simulink model "HVDC_VSC_1CPUcore_dcpl"  (Simulink 8.4)
settings: Solver=ode3  SolverMode=SingleTasking  StartTime=0.0  StopTime=70.0  FixedStep=Ts_Power  RelTol=1e-3  AbsTol=1e-2
PreLoadFcn:
  | Ts_Power=50e-6; Ts_Control=1*Ts_Power; init_cosim_IA; startup_transients_hvdc_vsc;
PostLoadFcn:
  | Ts_Power=50e-6; Ts_Control=1*Ts_Power; init_cosim_IA; startup_transients_hvdc_vsc;
InitFcn:
  | Ts_Power=50e-6; Ts_Control=1*Ts_Power; init_cosim_IA; startup_transients_hvdc_vsc;
values from neighbouring files (symbols this model uses):
  h = 5    [init_cosim_IA.m]
  intfDelay = 400.0    (= 400)    [init_cosim_IA.m]
  Ts_intf = 2*Ts_Power    [init_cosim_IA.m]
undefined symbols (not defined in the file or in its folder): CLARK, D1, Delta, dPref1_2, dPref1_2_rlimit, gcbh, level, lib_mesures, magnitude, ResistanceM, rte_drive_private_lib, rte_tsb3level_hiz_rect_cb, sps_rtmsupport, t_deblock_Pref1, t_deblock_Udref2, t_dPref1_2, t_init_AC, t_SwitchITMIdc, t_SwitchITMVdc, t_vsag_end, t_vsag_start, TSB3_hiZR
libraries: powerlib x162, powerlib_extras x71, spsVIMeasurementModel x63, rteventslib x26, op_dpl_lib x14, powerlib_meascontrol x14, rtlab x6, sps_avr x3, artemis x1
(part 7 of 11)

== system HVDC_VSC_1CPUcore_dcpl/SM_HVDC_VSC/VSC Controller (Station 2)/Discrete VSC Controller (Station 2)/Outer Active-Reactive Power and Voltage Loop ==
  note: Outer Active-Reactive Power and Voltage Loop
  Udc_meas : Inport
  Uf_meas : Inport  Port=2
  P_meas : Inport  Port=3
  Q_meas : Inport  Port=4
  U_meas : Inport  Port=5
  Pref : Inport  Port=6
  dPref : Inport  Port=7
  Qref : Inport  Port=8
  Udref : Inport  Port=9
  block_status : Inport  Port=10
  Active_Power_Control : Subsystem
  Constant19 : Constant  Value=Ki_dcvc
  Constant20 : Constant  Value=Kp_dcvc
  Constant9 : Constant  Value=P_control
  Current_Reference_Calculation : Subsystem
  Current_Reference_Limitation : Subsystem
  DC_Voltage_Control : Subsystem  TreatAsAtomicUnit=on
  Logical Operator1 : Logic  AllPortsSameDT=off
  Logical Operator4 : Logic  Operator=NOT  AllPortsSameDT=off
  Logical Operator6 : Logic  AllPortsSameDT=off
  Logical Operator7 : Logic  Operator=NOT  AllPortsSameDT=off
  Reactive_Power_Control : Subsystem
  Switch2 : Switch  Threshold=0.5  SaturateOnIntegerOverflow=on
  Iref_dq : Outport
  Pref_ramped : Outport  Port=2
  wires:
  Current_Reference_Limitation/1(Iref_dq) -> Iref_dq/1
  Switch2/1 -> Current_Reference_Limitation/1(Iref_d_tmp)
  Logical Operator4/1 -> Logical Operator1/1, Logical Operator6/2, Active_Power_Control/2(enable_ramp), Reactive_Power_Control/1(enable_control)
  Current_Reference_Calculation/1(Iref_d_crc) -> Switch2/1
  Constant20/1 -> DC_Voltage_Control/4(Kp_dcvc)
  Constant19/1 -> DC_Voltage_Control/3(Ki_dcvc)
  Q_meas/1 -> Reactive_Power_Control/3(Q_meas)
  P_meas/1 -> Active_Power_Control/5(P_meas)
  DC_Voltage_Control/1(Iref_d_dcvc) -> Switch2/3
  Udc_meas/1 -> Active_Power_Control/7(Udc_meas), DC_Voltage_Control/2(Udc_meas)
  block_status/1 -> Logical Operator4/1
  Constant9/1 -> Logical Operator6/1, Current_Reference_Limitation/3(P_control), Logical Operator7/1
  Logical Operator6/1 -> Switch2/2, Active_Power_Control/1(enable_control)
  U_meas/1 -> Reactive_Power_Control/4(U_meas), Active_Power_Control/6(U_meas)
  Current_Reference_Calculation/2(Iref_q_crc) -> Current_Reference_Limitation/2(Iref_q_tmp)
  dPref/1 -> Active_Power_Control/4(dPref)
  Active_Power_Control/1(Pref_apc) -> Current_Reference_Calculation/1(Pref_apc)
  Reactive_Power_Control/1(Qref_rpc) -> Current_Reference_Calculation/2(Qref_rpc)
  Pref/1 -> Active_Power_Control/3(Pref)
  Uf_meas/1 -> Current_Reference_Calculation/3(Uf_meas)
  Qref/1 -> Reactive_Power_Control/2(Qref)
  Logical Operator7/1 -> Logical Operator1/2
  Logical Operator1/1 -> DC_Voltage_Control/Enable
  Udref/1 -> DC_Voltage_Control/1(Udref)
  Active_Power_Control/2(Pref_ramped) -> Pref_ramped/1

== system HVDC_VSC_1CPUcore_dcpl/SM_HVDC_VSC/VSC Controller (Station 2)/Discrete VSC Controller (Station 2)/PLL ==
  note: Discrete 3-phase PLL
  note: Pierre Giroux, Gilbert Sybille
      | Power System Laboratory, IREQ
      | Hydro-Quebec
  U_AB : Inport
  Constant1 : Constant  Value=0
  Constant4 : Constant  Value=2*pi
  Discrete PI Controller : powerlib_extras/Discrete  Control Blocks/Discrete PI Controller  Kp=Kp  Ki=Ki  Par_Limits=2*pi*Finit*[1.25 0.75]  Init=2*pi*Finit  Ts=Ts
  Discrete Rate Limiter : powerlib_extras/Discrete  Control Blocks/Discrete Rate Limiter  R=12  F=-12  Vinit=Finit  Ts=Ts
  Discrete Variable Frequency Mean value : powerlib_extras/Discrete Measurements/Discrete Variable Frequency Mean value  Finit=Finit  Fmin=Fmin  Vinit=0  Ts=Ts
  Discrete  2nd-Order Filter : powerlib_extras/Discrete  Control Blocks/Discrete  2nd-Order Filter  FilterType=Lowpass  Fo=25  Zeta=0.707  Ts=Ts  Initialize=on  Vac_Init=[0 0 Finit]  Vdc_Init=Finit  PlotResponse=off  param1=[1 500 0.1]
  Discrete-Time Integrator : DiscreteIntegrator  InitialCondition=Phase_Init*pi/180  SampleTime=Ts
  Gain10 : Gain  Gain=1/2/pi  SaturateOnIntegerOverflow=on  OutDataTypeStr=Inherit: Same as input  ParamDataTypeStr=Inherit: Same as input
  Math Function : Math  Operator=mod  SaturateOnIntegerOverflow=on
  Mux1 : Mux  Inputs=[2 1]
  Mux2 : Mux  Inputs=2
  Selector : Selector  InputPortWidth=3  Indices=2
  Trigonometric Function : Trigonometry
  Trigonometric Function2 : Trigonometry  Operator=cos
  Unit Delay : UnitDelay  InitialCondition=Finit  SampleTime=Ts
  "ab0->dq0 " : Subsystem  AncestorBlock=lib_mesures/CLARK
  Freq : Outport
  theta : Outport  Port=2
  Sin_Cos : Outport  Port=3
  wires:
  Constant1/1 -> Mux1/2
  Mux1/1 -> "ab0->dq0 "/1(ab0)
  U_AB/1 -> Mux1/1
  Discrete Variable Frequency Mean value/1 -> Discrete PI Controller/1
  "ab0->dq0 "/1(dq0) -> Selector/1
  Constant4/1 -> Math Function/2
  Discrete-Time Integrator/1 -> Math Function/1
  Math Function/1 -> Trigonometric Function/1, Trigonometric Function2/1, theta/1
  Trigonometric Function/1 -> Mux2/1
  Trigonometric Function2/1 -> Mux2/2
  Mux2/1 -> "ab0->dq0 "/2(sin_cos), Sin_Cos/1
  Discrete PI Controller/1 -> Discrete-Time Integrator/1, Gain10/1  "W"
  Gain10/1 -> Discrete Rate Limiter/1
  Discrete Rate Limiter/1 -> Discrete  2nd-Order Filter/1
  Unit Delay/1 -> Freq/1, Discrete Variable Frequency Mean value/1
  Discrete  2nd-Order Filter/1 -> Unit Delay/1
  Selector/1 -> Discrete Variable Frequency Mean value/2  "Vq"

== system HVDC_VSC_1CPUcore_dcpl/SM_HVDC_VSC/VSC Controller (Station 2)/Discrete VSC Controller (Station 2)/Signal Calculations ==
  U_AB : Inport
  I_AB : Inport  Port=2
  Uf_AB : Inport  Port=3
  Vref_lim_AB : Inport  Port=4
  Udc_pn : Inport  Port=5
  Idc_pn : Inport  Port=6
  Freq : Inport  Port=7
  2nd-Order Filter : powerlib_extras/Discrete  Control Blocks/Discrete  2nd-Order Filter  FilterType=Lowpass  Fo=f0_sc  Zeta=zeta_sc  Ts=Ts_Control  Initialize=off  Vac_Init=[0.8 -25 60]  Vdc_Init=-0.4  PlotResponse=off  param1=[1 500 1]
  2nd-Order Filter2 : powerlib_extras/Discrete  Control Blocks/Discrete  2nd-Order Filter  FilterType=Lowpass  Fo=f0_sc  Zeta=zeta_sc  Ts=Ts_Control  Initialize=off  Vac_Init=[0.8 -25 60]  Vdc_Init=-0.4  PlotResponse=off  param1=[1 500 1]
  "2nd-Order Filter " : powerlib_extras/Discrete  Control Blocks/Discrete  2nd-Order Filter  FilterType=Lowpass  Fo=f0_sc  Zeta=zeta_sc  Ts=Ts_Control  Initialize=off  Vac_Init=[0.8 -25 60]  Vdc_Init=-0.4  PlotResponse=off  param1=[1 500 1]
  "2nd-Order Filter  " : powerlib_extras/Discrete  Control Blocks/Discrete  2nd-Order Filter  FilterType=Lowpass  Fo=f0_sc  Zeta=zeta_sc  Ts=Ts_Control  Initialize=off  Vac_Init=[0.8 -25 60]  Vdc_Init=-0.4  PlotResponse=off  param1=[1 500 1]
  2nd-Order Filter 1\ : powerlib_extras/Discrete  Control Blocks/Discrete  2nd-Order Filter  FilterType=Lowpass  Fo=f0_sc  Zeta=zeta_sc  Ts=Ts_Control  Initialize=off  Vac_Init=[0.8 -25 60]  Vdc_Init=-0.4  PlotResponse=off  param1=[1 500 1]
  Active_Power : Subsystem
  DC_Current : Subsystem
  DC_Voltage : Subsystem
  Demux : Demux  Outputs=2
  Demux1 : Demux  Outputs=2
  Filter_Bus_Voltage : Subsystem
  Gain1 : Gain  Gain=k_pu2nom_Vdc*k_pu2nom_Idc  SaturateOnIntegerOverflow=on  OutDataTypeStr=Inherit: Same as input  ParamDataTypeStr=Inherit: Same as input
  Modulation_Index : Subsystem
  PCC_Voltage : Subsystem
  Product5 : Product  SaturateOnIntegerOverflow=on  OutDataTypeStr=Inherit: Same as first input
  Reactive_Power : Subsystem
  Variable Frequency Mean value IC: 0 : powerlib_extras/Discrete Measurements/Discrete Variable Frequency Mean value  Finit=50  Fmin=f_min_pll  Vinit=0  Ts=Ts_Control
  Pdc_meas : Outport
  Mod_index : Outport  Port=2
  Udc_meas : Outport  Port=3
  Uf_meas : Outport  Port=4
  P_meas : Outport  Port=5
  Q_meas : Outport  Port=6
  U_meas : Outport  Port=7
  wires:
  Gain1/1 -> Pdc_meas/1
  Freq/1 -> Variable Frequency Mean value IC: 0/1
  Product5/1 -> Gain1/1
  Variable Frequency Mean value IC: 0/1 -> Product5/2
  2nd-Order Filter 1\/1 -> Uf_meas/1
  "2nd-Order Filter "/1 -> Mod_index/1
  Filter_Bus_Voltage/1(Uf_meas) -> 2nd-Order Filter 1\/1
  PCC_Voltage/1(Upcc) -> "2nd-Order Filter  "/1
  "2nd-Order Filter  "/1 -> U_meas/1
  Active_Power/1(Ppcc) -> 2nd-Order Filter/1
  2nd-Order Filter/1 -> P_meas/1
  Reactive_Power/1(Qpcc) -> 2nd-Order Filter2/1
  2nd-Order Filter2/1 -> Q_meas/1
  Modulation_Index/1(Mod_index) -> "2nd-Order Filter "/1
  Demux/2 -> DC_Voltage/2(Udc_n)
  Uf_AB/1 -> Filter_Bus_Voltage/1(Uf_AB)
  U_AB/1 -> PCC_Voltage/1(U_AB), Active_Power/1(U_AB), Reactive_Power/1(U_AB)
  I_AB/1 -> Active_Power/2(I_AB), Reactive_Power/2(I_AB)
  DC_Voltage/1(Udc_meas) -> Product5/1, Udc_meas/1, Modulation_Index/2(Udc_meas)
  DC_Current/1(Idc_meas) -> Variable Frequency Mean value IC: 0/2
  Udc_pn/1 -> Demux/1
  Demux/1 -> DC_Voltage/1(Udc_p)
  Demux1/1 -> DC_Current/1(Idc_p)
  Demux1/2 -> DC_Current/2(Idc_n)
  Idc_pn/1 -> Demux1/1
  Vref_lim_AB/1 -> Modulation_Index/1(Vref_lim_AB)

== system HVDC_VSC_1CPUcore_dcpl/SM_HVDC_VSC/VSC Controller (Station 2)/Discrete VSC Controller (Station 2)/dq  Transformations ==
  note: dq Transformations
  U_AB : Inport
  Iv_AB : Inport  Port=2
  sin_cos : Inport  Port=3
  Constant1 : Constant  Value=0
  Mux1 : Mux  Inputs=[2 1]
  Mux4 : Mux  Inputs=[2 1]
  Selector : Selector  InputPortWidth=3  Indices=[1 2]
  Selector3 : Selector  InputPortWidth=3  Indices=[1 2]
  ab0_to_dq0 : Subsystem  AncestorBlock=lib_mesures/CLARK
  "ab0_to_dq0   " : Subsystem  AncestorBlock=lib_mesures/CLARK
  U_dq : Outport
  Iv_dq : Outport  Port=2
  wires:
  Constant1/1 -> Mux4/2, Mux1/2
  Mux4/1 -> "ab0_to_dq0   "/1(ab0)
  Iv_AB/1 -> Mux4/1
  Mux1/1 -> ab0_to_dq0/1(ab0)
  U_AB/1 -> Mux1/1
  "ab0_to_dq0   "/1(dq0) -> Selector3/1
  ab0_to_dq0/1(dq0) -> Selector/1
  sin_cos/1 -> "ab0_to_dq0   "/2(sin_cos), ab0_to_dq0/2(sin_cos)
  Selector/1 -> U_dq/1
  Selector3/1 -> Iv_dq/1

== system HVDC_VSC_1CPUcore_dcpl/SM_HVDC_VSC/VSC Controller (Station 1)/Discrete VSC Controller (Station 1)/Clark Transformations/CLARK  ==
  note: CLARK transformation
  abc : Inport
  Fcn1 : Fcn  Expr=1/sqrt(3)*(u[2] - u[3])
  Fcn2 : Fcn  Expr=1/3*(2*u[1] - u[2] - u[3])
  Fcn3 : Fcn  Expr=1/3*(u[1] + u[2] + u[3])
  Mux : Mux  Inputs=3
  AB0 : Outport
  wires:
  Fcn2/1 -> Mux/1
  abc/1 -> Fcn1/1, Fcn3/1, Fcn2/1
  Fcn1/1 -> Mux/2
  Fcn3/1 -> Mux/3
  Mux/1 -> AB0/1

== system HVDC_VSC_1CPUcore_dcpl/SM_HVDC_VSC/VSC Controller (Station 1)/Discrete VSC Controller (Station 1)/Clark Transformations/CLARK   ==
  note: CLARK transformation
  abc : Inport
  Fcn1 : Fcn  Expr=1/sqrt(3)*(u[2] - u[3])
  Fcn2 : Fcn  Expr=1/3*(2*u[1] - u[2] - u[3])
  Fcn3 : Fcn  Expr=1/3*(u[1] + u[2] + u[3])
  Mux : Mux  Inputs=3
  AB0 : Outport
  wires:
  Mux/1 -> AB0/1
  Fcn3/1 -> Mux/3
  Fcn1/1 -> Mux/2
  abc/1 -> Fcn2/1, Fcn3/1, Fcn1/1
  Fcn2/1 -> Mux/1

== system HVDC_VSC_1CPUcore_dcpl/SM_HVDC_VSC/VSC Controller (Station 1)/Discrete VSC Controller (Station 1)/Clark Transformations/CLARK_YD ==
  note: Rotation of pi/6
  note: Rotation of - pi/6
  note: Transformer Connexion:
      | YY = 0
      | YD1 (laging) = 1
      | YD11 (leading)= 2
  note: CLARK transformation
  abc : Inport
  Tr_conx : Inport  Port=2
  CLARK : Subsystem  AncestorBlock=lib_mesures/CLARK  TreatAsAtomicUnit=on
  CLARK_YD1 : Subsystem  AncestorBlock=lib_mesures/CLARK  TreatAsAtomicUnit=on
  CLARK_YD11 : Subsystem  AncestorBlock=lib_mesures/CLARK  TreatAsAtomicUnit=on
  Constant : Constant  Value=2
  Constant1 : Constant  Value=0
  Constant2 : Constant
  Relational Operator1 : RelationalOperator  Operator===  InputSameDT=on
  Relational Operator2 : RelationalOperator  Operator===  InputSameDT=on
  Relational Operator3 : RelationalOperator  Operator===  InputSameDT=on
  Sum : Sum  Inputs=+++  SaturateOnIntegerOverflow=on
  AB0 : Outport
  wires:
  Constant2/1 -> Relational Operator3/2
  Relational Operator2/1 -> CLARK/Enable
  Constant1/1 -> Relational Operator2/2
  CLARK/1(AB0) -> Sum/3
  Sum/1 -> AB0/1
  CLARK_YD1/1(AB0) -> Sum/2
  CLARK_YD11/1(AB0) -> Sum/1
  abc/1 -> CLARK/1(abc), CLARK_YD1/1(abc), CLARK_YD11/1(abc)
  Relational Operator1/1 -> CLARK_YD11/Enable
  Relational Operator3/1 -> CLARK_YD1/Enable
  Tr_conx/1 -> Relational Operator3/1, Relational Operator2/1, Relational Operator1/1
  Constant/1 -> Relational Operator1/2

== system HVDC_VSC_1CPUcore_dcpl/SM_HVDC_VSC/VSC Controller (Station 1)/Discrete VSC Controller (Station 1)/Clark Transformations/CLARK_YD  ==
  note: CLARK transformation
  note: Transformer Connexion:
      | YY = 0
      | YD1 (laging) = 1
      | YD11 (leading)= 2
  note: Rotation of - pi/6
  note: Rotation of pi/6
  abc : Inport
  Tr_conx : Inport  Port=2
  CLARK : Subsystem  AncestorBlock=lib_mesures/CLARK  TreatAsAtomicUnit=on
  CLARK_YD1 : Subsystem  AncestorBlock=lib_mesures/CLARK  TreatAsAtomicUnit=on
  CLARK_YD11 : Subsystem  AncestorBlock=lib_mesures/CLARK  TreatAsAtomicUnit=on
  Constant : Constant  Value=2
  Constant1 : Constant  Value=0
  Constant2 : Constant
  Relational Operator1 : RelationalOperator  Operator===  InputSameDT=on
  Relational Operator2 : RelationalOperator  Operator===  InputSameDT=on
  Relational Operator3 : RelationalOperator  Operator===  InputSameDT=on
  Sum : Sum  Inputs=+++  SaturateOnIntegerOverflow=on
  AB0 : Outport
  wires:
  Constant/1 -> Relational Operator1/2
  Tr_conx/1 -> Relational Operator1/1, Relational Operator2/1, Relational Operator3/1
  Relational Operator3/1 -> CLARK_YD1/Enable
  Relational Operator1/1 -> CLARK_YD11/Enable
  abc/1 -> CLARK_YD11/1(abc), CLARK_YD1/1(abc), CLARK/1(abc)
  CLARK_YD11/1(AB0) -> Sum/1
  CLARK_YD1/1(AB0) -> Sum/2
  Sum/1 -> AB0/1
  CLARK/1(AB0) -> Sum/3
  Constant1/1 -> Relational Operator2/2
  Relational Operator2/1 -> CLARK/Enable
  Constant2/1 -> Relational Operator3/2

== system HVDC_VSC_1CPUcore_dcpl/SM_HVDC_VSC/VSC Controller (Station 1)/Discrete VSC Controller (Station 1)/DC Voltage Balance Control/Regulator ==
  note: Reset states when enabling
  note: Voltage Sign
  note: Reversed Current Sign
  V_ref_lim_abc : Inport
  Iv_abc : Inport  Port=2
  Udc_0_mean : Inport  Port=3
  Enable : EnablePort  StatesWhenEnabling=reset
  Constant1 : Constant  Value=0
  Constant13 : Constant  Value=Ki_dcvbc
  Constant2 : Constant  Value=0
  Constant3 : Constant  Value=-1
  Constant4 : Constant
  Constant5 : Constant
  Constant6 : Constant  Value=-1
  Constant7 : Constant  Value=0
  Constant8 : Constant  Value=Kp_dcvbc
  "PI_regulator " : Subsystem  mask(PI regulator - type 2){max_i=max_out_dcvbc, min_i=min_out_dcvbc, i_ic=0, max_out=max_out_dcvbc, min_out=min_out_dcvbc, Ts=Ts_Control}
      mask prompts: max_i "Integrator maximum  limit:"; min_i "Integrator minimum  limit:"; i_ic "Integrator initial condition:"; max_out "Output maximum limit:"; min_out "Output minimum limit:"; Ts "Sample time: (s)"
  Product : Product  Inputs=3  SaturateOnIntegerOverflow=on  OutDataTypeStr=Inherit: Same as first input
  Relational Operator : RelationalOperator  Operator=<
  Relational Operator1 : RelationalOperator  Operator=<
  Switch : Switch  Threshold=0.5  SaturateOnIntegerOverflow=on
  Switch1 : Switch  Threshold=0.5  SaturateOnIntegerOverflow=on
  dV_ref_abc_dcvbc : Outport
  wires:
  Switch1/1 -> Product/2
  Constant1/1 -> "PI_regulator "/5(Kf), "PI_regulator "/2(Meas)
  Constant13/1 -> "PI_regulator "/3(Ki)
  Constant8/1 -> "PI_regulator "/4(Kp)
  "PI_regulator "/1(Out) -> Product/3
  Constant2/1 -> Relational Operator/2
  Constant3/1 -> Switch/1
  Constant4/1 -> Switch/3
  Relational Operator/1 -> Switch/2
  Constant5/1 -> Switch1/1
  Constant6/1 -> Switch1/3
  Relational Operator1/1 -> Switch1/2
  Switch/1 -> Product/1
  V_ref_lim_abc/1 -> Relational Operator/1
  Product/1 -> dV_ref_abc_dcvbc/1
  Iv_abc/1 -> Relational Operator1/1
  Udc_0_mean/1 -> "PI_regulator "/1(Ord)
  Constant7/1 -> Relational Operator1/2

== system HVDC_VSC_1CPUcore_dcpl/SM_HVDC_VSC/VSC Controller (Station 1)/Discrete VSC Controller (Station 1)/Inner Current Loop/AC_Current_Control ==
  note: Uq
  note: Ud
  note: AC Current Control
  note: d axis
  note: q axis
  Iv_dq : Inport
  Iref_dq : Inport  Port=2
  U_dq : Inport  Port=3
  Freq : Inport  Port=4
  Constant1 : Constant  Value=Kp_accc
  Constant13 : Constant  Value=Ki_accc
  Constant2 : Constant  Value=1.0
  Constant3 : Constant  Value=Kf_accc
  Demux : Demux  Outputs=2
  Demux1 : Demux  Outputs=2
  Demux2 : Demux  Outputs=2
  IC: 1.0 : powerlib_extras/Discrete Measurements/Discrete Variable Frequency Mean value  Finit=60  Fmin=f_min_pll  Vinit=1.0  Ts=Ts_Control
  Mux : Mux  Inputs=2
  "PI_regulator " : Subsystem  mask(PI regulator - type 2){max_i=max_out_accc, min_i=min_out_accc, i_ic=0, max_out=max_out_accc, min_out=min_out_accc, Ts=Ts_Control}
      mask prompts: max_i "Integrator maximum  limit:"; min_i "Integrator minimum  limit:"; i_ic "Integrator initial condition:"; max_out "Output maximum limit:"; min_out "Output minimum limit:"; Ts "Sample time: (s)"
  PI_regulator_2 : Subsystem  mask(PI regulator - type 2){max_i=max_out_accc, min_i=min_out_accc, i_ic=0, max_out=max_out_accc, min_out=min_out_accc, Ts=Ts_Control}
      mask prompts: max_i "Integrator maximum  limit:"; min_i "Integrator minimum  limit:"; i_ic "Integrator initial condition:"; max_out "Output maximum limit:"; min_out "Output minimum limit:"; Ts "Sample time: (s)"
  Product : Product  SaturateOnIntegerOverflow=on  OutDataTypeStr=Inherit: Same as first input
  Product1 : Product  SaturateOnIntegerOverflow=on  OutDataTypeStr=Inherit: Same as first input
  Sum2 : Sum  Inputs=+|-|+  SaturateOnIntegerOverflow=on  InputSameDT=on  OutDataTypeStr=Inherit: Same as first input
  Sum3 : Sum  Inputs=--+  SaturateOnIntegerOverflow=on  InputSameDT=on  OutDataTypeStr=Inherit: Same as first input
  "Variable Frequency Mean value IC:1.0 " : powerlib_extras/Discrete Measurements/Discrete Variable Frequency Mean value  Finit=60  Fmin=f_min_pll  Vinit=1.0  Ts=Ts_Control
  Vref_dq_tmp : Outport
  wires:
  Constant3/1 -> Product1/1, Product/2
  Sum3/1 -> Mux/2
  IC: 1.0/1 -> Sum3/3
  Demux2/2 -> IC: 1.0/2
  Product1/1 -> Sum3/2
  Sum2/1 -> Mux/1
  "Variable Frequency Mean value IC:1.0 "/1 -> Sum2/1
  Freq/1 -> IC: 1.0/1, "Variable Frequency Mean value IC:1.0 "/1
  Demux2/1 -> "Variable Frequency Mean value IC:1.0 "/2
  Product/1 -> Sum2/3
  PI_regulator_2/1(Out) -> Sum3/1
  "PI_regulator "/1(Out) -> Sum2/2
  Iref_dq/1 -> Demux1/1
  Iv_dq/1 -> Demux/1
  Demux1/1 -> "PI_regulator "/1(Ord)  "I_ref_d"
  Demux/1 -> Product1/2, "PI_regulator "/2(Meas)  "Iv_d"
  Constant2/1 -> "PI_regulator "/5(Kf), PI_regulator_2/5(Kf)
  Demux/2 -> Product/1, PI_regulator_2/2(Meas)  "Iv_q"
  Constant13/1 -> "PI_regulator "/3(Ki), PI_regulator_2/3(Ki)
  Mux/1 -> Vref_dq_tmp/1
  Constant1/1 -> "PI_regulator "/4(Kp), PI_regulator_2/4(Kp)
  Demux1/2 -> PI_regulator_2/1(Ord)  "I_ref_q"
  U_dq/1 -> Demux2/1

== system HVDC_VSC_1CPUcore_dcpl/SM_HVDC_VSC/VSC Controller (Station 1)/Discrete VSC Controller (Station 1)/Inner Current Loop/Inverse_Clark ==
  note: Inverse CLARK transformation
  AB0 : Inport
  Fcn1 : Fcn  Expr="1/2*(-u[1]  + sqrt(3)*u[2] + 2*u[3])"
  Fcn2 : Fcn  Expr=(u[1] - u[3])
  Fcn3 : Fcn  Expr=1/2*(-u[1] - sqrt(3)*u[2] + 2*u[3])
  Mux : Mux  Inputs=3
  abc : Outport
  wires:
  Fcn2/1 -> Mux/1
  AB0/1 -> Fcn1/1, Fcn3/1, Fcn2/1
  Fcn1/1 -> Mux/2
  Fcn3/1 -> Mux/3
  Mux/1 -> abc/1

== system HVDC_VSC_1CPUcore_dcpl/SM_HVDC_VSC/VSC Controller (Station 1)/Discrete VSC Controller (Station 1)/Inner Current Loop/Reference_Voltage_Conditioning ==
  note: Maximum AC Voltage / DC Voltage (pole-neutral)
  note: Voltage Reference Conditioning
  Vref_dq_tmp : Inport
  Udc_meas_mean : Inport  Port=2
  Constant2 : Constant  Value=K_pwm
  Gain1 : Gain  Gain=k_pu2nom_Vdc  SaturateOnIntegerOverflow=on  OutDataTypeStr=Inherit: Same as input  ParamDataTypeStr=Inherit: Same as input
  Product1 : Product  Inputs=**/  SaturateOnIntegerOverflow=on  OutDataTypeStr=Inherit: Same as first input
  Vref_dq : Outport
  wires:
  Gain1/1 -> Product1/2
  Udc_meas_mean/1 -> Gain1/1
  Product1/1 -> Vref_dq/1
  Vref_dq_tmp/1 -> Product1/1
  Constant2/1 -> Product1/3

== system HVDC_VSC_1CPUcore_dcpl/SM_HVDC_VSC/VSC Controller (Station 1)/Discrete VSC Controller (Station 1)/Inner Current Loop/Reference_Voltage_Limitation ==
  note: Limitation on a circle of 1 p.u. radius
  note: Reference Voltage Limitation
  note: Not Limited
  note: Limited
  Vref_dq : Inport
  Constant2 : Constant  Value=1.0
  Math Function : Math  Operator=magnitude^2  SaturateOnIntegerOverflow=on
  Math Function1 : Math  Operator=sqrt  SaturateOnIntegerOverflow=on
  Max=inf Min=eps : Saturate  UpperLimit=1e6  LowerLimit=1e-6
  Product : Product  Inputs=/*  SaturateOnIntegerOverflow=on  OutDataTypeStr=Inherit: Same as first input
  Relational Operator1 : RelationalOperator  Operator=<
  Sum : Sum  Inputs=+  SaturateOnIntegerOverflow=on
  Switch : Switch  Threshold=0.5  SaturateOnIntegerOverflow=on
  Vref_lim_dq : Outport
  wires:
  Max=inf Min=eps/1 -> Product/1
  Relational Operator1/1 -> Switch/2
  Math Function1/1 -> Max=inf Min=eps/1, Relational Operator1/1
  Vref_dq/1 -> Math Function/1, Switch/1, Product/2
  Math Function/1 -> Sum/1
  Sum/1 -> Math Function1/1
  Product/1 -> Switch/3
  Switch/1 -> Vref_lim_dq/1
  Constant2/1 -> Relational Operator1/2

== system HVDC_VSC_1CPUcore_dcpl/SM_HVDC_VSC/VSC Controller (Station 1)/Discrete VSC Controller (Station 1)/Inner Current Loop/dq0 to abo ==
  note: X0 = X0
  note: dq0 to ab0
  note: Xa = Xd*sin(wt) + Xq*cos(wt)
  note: Xb = -Xd*cos(wt) + Xq*sin(wt)
  dq0 : Inport
  sin_cos : Inport  Port=2
  Demux : Demux  Outputs=2
  Demux1 : Demux  Outputs=3
  Mux : Mux  Inputs=3
  Product{,1..3} (4 alike) : Product  SaturateOnIntegerOverflow=on  InputSameDT=on  OutDataTypeStr=Inherit: Same as first input
  Sum1 : Sum  Inputs=+-  SaturateOnIntegerOverflow=on  InputSameDT=on  OutDataTypeStr=Inherit: Same as first input
  Sum4 : Sum  Inputs=2  SaturateOnIntegerOverflow=on  InputSameDT=on  OutDataTypeStr=Inherit: Same as first input
  ab0 : Outport
  wires:
  dq0/1 -> Demux1/1
  Mux/1 -> ab0/1
  Product3/1 -> Sum1/2
  Product2/1 -> Sum1/1
  Product1/1 -> Sum4/1
  Product/1 -> Sum4/2
  sin_cos/1 -> Demux/1
  Sum4/1 -> Mux/1
  Demux1/1 -> Product1/1, Product3/1
  Demux/1 -> Product1/2, Product2/2
  Demux/2 -> Product/2, Product3/2
  Demux1/2 -> Product/1, Product2/1
  Sum1/1 -> Mux/2
  Demux1/3 -> Mux/3

== system HVDC_VSC_1CPUcore_dcpl/SM_HVDC_VSC/VSC Controller (Station 1)/Discrete VSC Controller (Station 1)/Outer Active-Reactive Power and Voltage Loop/Active_Power_Control ==
  note: Active Power Control
  enable_control : Inport
  enable_ramp : Inport  Port=2
  Pref : Inport  Port=3
  dPref : Inport  Port=4
  P_meas : Inport  Port=5
  U_meas : Inport  Port=6
  Udc_meas : Inport  Port=7
  Constant1 : Constant  Value=Udc_max
  Constant11 : Constant  Value=Ki_apc
  Constant12 : Constant  Value=Ramp_apc
  Constant13 : Constant  Value=P_max
  Constant14 : Constant  Value=P_min
  Constant2 : Constant  Value=Udc_min
  Constant25 : Constant  Value=Ki_apc_vco
  Constant3 : Constant  Value=Kp_apc_vco
  DC Voltage Control Override : Subsystem  TreatAsAtomicUnit=on
  Freeze_integrator : Subsystem
  Max=P_max Min=P_min : Saturate  UpperLimit=P_max  LowerLimit=P_min
  Ramping : Subsystem
  Regulator : Subsystem  TreatAsAtomicUnit=on
  Sum1 : Sum  SaturateOnIntegerOverflow=on
  Sum2 : Sum  SaturateOnIntegerOverflow=on
  Pref_apc : Outport
  Pref_ramped : Outport  Port=2
  wires:
  U_meas/1 -> Freeze_integrator/1(U_meas)
  Freeze_integrator/1(Freeze) -> Regulator/6(Freeze)
  Constant14/1 -> Regulator/5(min_out)
  Constant13/1 -> Regulator/4(max_out)
  enable_ramp/1 -> Ramping/1(enable_ramp)
  Pref/1 -> Ramping/2(Pref)
  Constant12/1 -> Ramping/3(ramp_apc)
  P_meas/1 -> Regulator/2(Meas)
  Constant11/1 -> Regulator/3(Ki)
  Sum2/1 -> Regulator/1(Ord), Pref_ramped/1
  dPref/1 -> Sum2/2
  Ramping/1(Pref_ramp) -> Sum2/1
  enable_control/1 -> Regulator/Enable, DC Voltage Control Override/Enable
  Regulator/1(Out) -> Sum1/1
  Sum1/1 -> Max=P_max Min=P_min/1
  DC Voltage Control Override/1(Out) -> Sum1/2
  Constant25/1 -> DC Voltage Control Override/1(Ki_apc_vco)
  Constant1/1 -> DC Voltage Control Override/3(Udc_max)
  Constant2/1 -> DC Voltage Control Override/4(Udc_min)
  Udc_meas/1 -> DC Voltage Control Override/5(Udc_meas)
  Constant3/1 -> DC Voltage Control Override/2(Kp_apc_vco)
  Max=P_max Min=P_min/1 -> Pref_apc/1

== system HVDC_VSC_1CPUcore_dcpl/SM_HVDC_VSC/VSC Controller (Station 1)/Discrete VSC Controller (Station 1)/Outer Active-Reactive Power and Voltage Loop/Current_Reference_Calculation ==
  note: Current Reference Calculation
  Pref_apc : Inport
  Qref_rpc : Inport  Port=2
  Uf_meas : Inport  Port=3
  2nd-Order Filter : powerlib_extras/Discrete  Control Blocks/Discrete  2nd-Order Filter  FilterType=Lowpass  Fo=f0_crc  Zeta=1/sqrt(2)  Ts=Ts_Control  Initialize=off  Vac_Init=[0.8 -25 60]  Vdc_Init=-0.4  PlotResponse=off  param1=[1 500 1]
  Constant22 : Constant  Value=lim_d_crc
  Constant23 : Constant  Value=lim_q_crc
  Constant24 : Constant  Value=U_level_crc
  Gain1 : Gain  Gain=-1  SaturateOnIntegerOverflow=on  OutDataTypeStr=Inherit: Same as input  ParamDataTypeStr=Inherit: Same as input
  Gain2 : Gain  Gain=-1  SaturateOnIntegerOverflow=on  OutDataTypeStr=Inherit: Same as input  ParamDataTypeStr=Inherit: Same as input
  MinMax : MinMax  Function=max  Inputs=2  SaturateOnIntegerOverflow=on  InputSameDT=on
  Product : Product  Inputs=*/  SaturateOnIntegerOverflow=on  OutDataTypeStr=Inherit: Same as first input
  Product1 : Product  Inputs=/*  SaturateOnIntegerOverflow=on  OutDataTypeStr=Inherit: Same as first input
  S1 : Subsystem  AncestorBlock=|  mask(Limiter with External Limits){}
      | powerlib_extras/Discrete 
      | Control Blocks/Discrete 12-Pulse
      | HVDC Control /Functions
      | (Discrete)/Current Regulator/S16/S6
      mask Display: disp('      Limiter\n')
  S2 : Subsystem  AncestorBlock=|  mask(Limiter with External Limits){}
      | powerlib_extras/Discrete 
      | Control Blocks/Discrete 12-Pulse
      | HVDC Control /Functions
      | (Discrete)/Current Regulator/S16/S6
      mask Display: disp('      Limiter\n')
  sat : Saturate  UpperLimit=1e6  LowerLimit=1e-6
  Iref_d_crc : Outport
  Iref_q_crc : Outport  Port=2
  wires:
  2nd-Order Filter/1 -> MinMax/2
  S2/1("  ") -> Iref_q_crc/1
  S1/1("  ") -> Iref_d_crc/1
  Uf_meas/1 -> 2nd-Order Filter/1
  Constant24/1 -> MinMax/1
  Pref_apc/1 -> Product/1
  sat/1 -> Product/2, Product1/1
  Qref_rpc/1 -> Product1/2
  Product/1 -> S1/2(In)
  Product1/1 -> S2/2(In)
  Constant22/1 -> Gain1/1, S1/1(MAX)
  Gain1/1 -> S1/3(MIN)
  Constant23/1 -> Gain2/1, S2/1(MAX)
  Gain2/1 -> S2/3(MIN)
  MinMax/1 -> sat/1

== system HVDC_VSC_1CPUcore_dcpl/SM_HVDC_VSC/VSC Controller (Station 1)/Discrete VSC Controller (Station 1)/Outer Active-Reactive Power and Voltage Loop/Current_Reference_Limitation ==
  note: DC Voltage Control mode (Active power priority)
  note: Power Control mode (Equal scaling)
  note: Current Reference Limitation
  Iref_d_tmp : Inport  PortDimensions=1
  Iref_q_tmp : Inport  Port=2  PortDimensions=1
  P_control : Inport  Port=3
  Constant25 : Constant  Value=Iref_max
  Double click here for  info : Subsystem
      mask Display: disp('?')
  Math Function1 : Math  Operator=sqrt  SaturateOnIntegerOverflow=on
  Math Function2 : Math  Operator=magnitude^2  SaturateOnIntegerOverflow=on
  Math Function3 : Math  Operator=magnitude^2  SaturateOnIntegerOverflow=on
  Math Function4 : Math  Operator=magnitude^2  SaturateOnIntegerOverflow=on
  Math Function5 : Math  Operator=sqrt  SaturateOnIntegerOverflow=on
  Min:eps Max:inf : Saturate  UpperLimit=1e6  LowerLimit=1e-6
  Mux : Mux  Inputs=2
  Mux1 : Mux  Inputs=2
  Product1 : Product  SaturateOnIntegerOverflow=on  OutDataTypeStr=Inherit: Same as first input
  Product2 : Product  Inputs=*/  SaturateOnIntegerOverflow=on  OutDataTypeStr=Inherit: Same as first input
  Relational Operator1 : RelationalOperator
  Relational Operator3 : RelationalOperator
  Sign : Signum
  Sum : Sum  Inputs=+  SaturateOnIntegerOverflow=on
  Sum2 : Sum  Inputs=-+  SaturateOnIntegerOverflow=on
  Switch1 : Switch  Threshold=0.5  SaturateOnIntegerOverflow=on
  Switch2 : Switch  Threshold=0.5  SaturateOnIntegerOverflow=on
  Switch3 : Switch  Threshold=0.5  SaturateOnIntegerOverflow=on
  Iref_dq : Outport
  wires:
  Sign/1 -> Product1/2
  Math Function5/1 -> Product1/1
  Product1/1 -> Mux1/2
  Sum2/1 -> Math Function5/1
  Math Function4/1 -> Sum2/1
  Math Function3/1 -> Sum2/2
  Mux1/1 -> Switch2/3
  Switch1/1 -> Iref_dq/1
  Switch2/1 -> Switch1/1
  Product2/1 -> Switch2/1
  Min:eps Max:inf/1 -> Product2/2
  Relational Operator1/1 -> Switch1/2
  Constant25/1 -> Relational Operator3/2, Switch3/1, Math Function3/1, Relational Operator1/2
  Math Function1/1 -> Min:eps Max:inf/1, Relational Operator1/1
  Mux/1 -> Product2/1, Math Function2/1, Switch1/3
  Iref_q_tmp/1 -> Sign/1, Mux/2
  Iref_d_tmp/1 -> Relational Operator3/1, Switch3/3, Mux/1
  Sum/1 -> Math Function1/1
  Math Function2/1 -> Sum/1
  P_control/1 -> Switch2/2
  Relational Operator3/1 -> Switch3/2
  Switch3/1 -> Mux1/1, Math Function4/1

== system HVDC_VSC_1CPUcore_dcpl/SM_HVDC_VSC/VSC Controller (Station 1)/Discrete VSC Controller (Station 1)/Outer Active-Reactive Power and Voltage Loop/DC_Voltage_Control ==
  note: DC Voltage Control
  note: Reset integrator when enabling
  note: pu DC --> pu AC
  Udref : Inport
  Udc_meas : Inport  Port=2
  Ki_dcvc : Inport  Port=3
  Kp_dcvc : Inport  Port=4
  Enable : EnablePort  StatesWhenEnabling=reset
  Constant1 : Constant  Value=0
  Constant2 : Constant  Value=max_i_dcvc
  Constant3 : Constant  Value=min_i_dcvc
  Constant4 : Constant  Value=max_out_dcvc
  Constant5 : Constant
  Constant6 : Constant  Value=min_out_dcvc
  First-Order_LP f0_Udc IC= k_nom2pu_Vdc : powerlib_extras/Discrete  Control Blocks/Discrete 1st-Order Filter  FilterType=Lowpass  Tc=1/(2*pi*f0_Udc)  Ts=Ts_Control  Initialize=on  Vac_Init=[0 0 60]  Vdc_Init=k_nom2pu_Vdc  PlotResponse=off  param1=[1 600 0.1]
  Gain1 : Gain  Gain=k_nom2pu_Vdc  SaturateOnIntegerOverflow=on  OutDataTypeStr=Inherit: Same as input  ParamDataTypeStr=Inherit: Same as input
  Ic=0 : UnitDelay  SampleTime=Ts_Control
  Kf_dcvc : Constant  Value=1.0
  Logical Operator : Logic  Operator=NOT  Inputs=1  AllPortsSameDT=off
  PI : Subsystem  mask(Integrator  With  External  Dynamic  Limits (Discrete)){i_ic=0, Ts=Ts_Control}
      mask prompts: i_ic "Initial Condition:"; Ts "Sample time: (s)"
      mask Display: disp('Discrete-Time\n(Trapezoidal)\nIntegrator\n ')
  Product2 : Product  SaturateOnIntegerOverflow=on  OutDataTypeStr=Inherit: Same as first input
  Product3 : Product  SaturateOnIntegerOverflow=on  OutDataTypeStr=Inherit: Same as first input
  S6 : Subsystem  AncestorBlock=|  mask(Limiter with External Limits){}
      | powerlib_extras/Discrete 
      | Control Blocks/Discrete 12-Pulse
      | HVDC Control /Functions
      | (Discrete)/Current Regulator/S16/S6
      mask Display: disp('      Limiter\n')
  Sum1 : Sum  Inputs=+-  SaturateOnIntegerOverflow=on
  Sum2 : Sum  SaturateOnIntegerOverflow=on
  Sum3 : Sum  Inputs=|+-  SaturateOnIntegerOverflow=on
  Sum4 : Sum  SaturateOnIntegerOverflow=on
  Iref_d_dcvc : Outport
  wires:
  Product3/1 -> Sum2/1
  Kp_dcvc/1 -> Product3/1
  Logical Operator/1 -> PI/5(Hold), PI/6(Reset)
  Constant5/1 -> Logical Operator/1
  Constant1/1 -> PI/7(Reset Value)
  Constant3/1 -> PI/2(Min)
  Constant2/1 -> PI/1(Max)
  Constant6/1 -> S6/3(MIN)
  Constant4/1 -> S6/1(MAX)
  Sum2/1 -> S6/2(In), Sum3/2
  Sum1/1 -> Product3/2, Sum4/1
  PI/1(Out) -> Sum2/2
  Udc_meas/1 -> First-Order_LP f0_Udc IC= k_nom2pu_Vdc/1
  Ki_dcvc/1 -> PI/4(Ki)
  S6/1("  ") -> Sum3/1, Iref_d_dcvc/1
  Sum4/1 -> PI/3(In)
  Ic=0/1 -> Sum4/2
  Sum3/1 -> Product2/2
  Product2/1 -> Ic=0/1
  Kf_dcvc/1 -> Product2/1
  First-Order_LP f0_Udc IC= k_nom2pu_Vdc/1 -> Sum1/2
  Udref/1 -> Gain1/1
  Gain1/1 -> Sum1/1

== system HVDC_VSC_1CPUcore_dcpl/SM_HVDC_VSC/VSC Controller (Station 1)/Discrete VSC Controller (Station 1)/Outer Active-Reactive Power and Voltage Loop/Reactive_Power_Control ==
  note: Reactive Power Control
  enable_control : Inport
  Qref : Inport  Port=2
  Q_meas : Inport  Port=3
  U_meas : Inport  Port=4
  AC Voltage Control Override : Subsystem  TreatAsAtomicUnit=on
  Constant1 : Constant  Value=U_max
  Constant2 : Constant  Value=U_min
  Constant25 : Constant  Value=Ki_rpc_vco
  Constant3 : Constant  Value=Kp_rpc_vco
  Constant4 : Constant  Value=Ki_rpc
  Constant5 : Constant  Value=Q_max
  Constant6 : Constant  Value=Q_min
  Freeze_integrator : Subsystem
  Max=Q_max Min=Q_min : Saturate  UpperLimit=Q_max  LowerLimit=Q_min
  Regulator : Subsystem  TreatAsAtomicUnit=on
  Sum2 : Sum  SaturateOnIntegerOverflow=on
  Qref_rpc : Outport
  wires:
  Sum2/1 -> Max=Q_max Min=Q_min/1
  Regulator/1(Out) -> Sum2/1
  Qref/1 -> Regulator/1(Ord)
  Constant5/1 -> Regulator/4(max_out)
  Constant6/1 -> Regulator/5(min_out)
  Constant4/1 -> Regulator/3(Ki)
  Q_meas/1 -> Regulator/2(Meas)
  U_meas/1 -> AC Voltage Control Override/5(U_meas), Freeze_integrator/1(U_meas)
  enable_control/1 -> Regulator/Enable, AC Voltage Control Override/Enable
  Constant25/1 -> AC Voltage Control Override/1(Ki_rpc_vco)
  Constant3/1 -> AC Voltage Control Override/2(Kp_rpc_vco)
  Constant1/1 -> AC Voltage Control Override/3(U_max)
  Constant2/1 -> AC Voltage Control Override/4(U_min)
  AC Voltage Control Override/1(Out) -> Sum2/2
  Max=Q_max Min=Q_min/1 -> Qref_rpc/1
  Freeze_integrator/1(Freeze) -> Regulator/6(freeze)

== system HVDC_VSC_1CPUcore_dcpl/SM_HVDC_VSC/VSC Controller (Station 1)/Discrete VSC Controller (Station 1)/PLL/ab0->dq0  ==
  note: Xq = Xa*cos(wt) + Xb*sin(wt)
  note: Xd = Xa*sin(wt) - Xb*cos(wt)
  note: Alpha-Beta-zero to dq0
  note: X0 = X0
  ab0 : Inport
  sin_cos : Inport  Port=2
  Demux : Demux  Outputs=2
  Demux1 : Demux  Outputs=3
  Mux : Mux  Inputs=3
  Product{,1..3} (4 alike) : Product  SaturateOnIntegerOverflow=on  InputSameDT=on  OutDataTypeStr=Inherit: Same as first input
  Sum1 : Sum  Inputs=+-  SaturateOnIntegerOverflow=on  InputSameDT=on  OutDataTypeStr=Inherit: Same as first input
  Sum4 : Sum  Inputs=2  SaturateOnIntegerOverflow=on  InputSameDT=on  OutDataTypeStr=Inherit: Same as first input
  dq0 : Outport
  wires:
  Sum4/1 -> Mux/2
  Sum1/1 -> Mux/1
  sin_cos/1 -> Demux/1
  Demux/2 -> Product/2, Product3/2
  Demux1/1 -> Product/1, Product2/1
  Product/1 -> Sum4/2
  Demux/1 -> Product2/2, Product1/2
  Demux1/2 -> Product1/1, Product3/1
  Product1/1 -> Sum4/1
  Product2/1 -> Sum1/1
  Product3/1 -> Sum1/2
  Mux/1 -> dq0/1
  ab0/1 -> Demux1/1
  Demux1/3 -> Mux/3

== system HVDC_VSC_1CPUcore_dcpl/SM_HVDC_VSC/VSC Controller (Station 1)/Discrete VSC Controller (Station 1)/Signal Calculations/Active_Power ==
  note: Active Power Calculation
  U_AB : Inport
  I_AB : Inport  Port=2
  Demux : Demux  Outputs=2
  Demux1 : Demux  Outputs=2
  Product : Product  SaturateOnIntegerOverflow=on  OutDataTypeStr=Inherit: Same as first input
  Product1 : Product  SaturateOnIntegerOverflow=on  OutDataTypeStr=Inherit: Same as first input
  Sum : Sum  SaturateOnIntegerOverflow=on
  Ppcc : Outport
  wires:
  U_AB/1 -> Demux/1
  I_AB/1 -> Demux1/1
  Demux/1 -> Product/1
  Demux1/1 -> Product/2
  Demux/2 -> Product1/1
  Demux1/2 -> Product1/2
  Product/1 -> Sum/1
  Product1/1 -> Sum/2
  Sum/1 -> Ppcc/1

== system HVDC_VSC_1CPUcore_dcpl/SM_HVDC_VSC/VSC Controller (Station 1)/Discrete VSC Controller (Station 1)/Signal Calculations/DC_Current ==
  note: DC Current Calculation
  Idc_p : Inport
  Idc_n : Inport  Port=2
  Gain : Gain  Gain=0.5  SaturateOnIntegerOverflow=on  OutDataTypeStr=Inherit: Same as input  ParamDataTypeStr=Inherit: Same as input
  Sum : Sum  Inputs=+-  SaturateOnIntegerOverflow=on
  Idc_meas : Outport
  wires:
  Gain/1 -> Idc_meas/1
  Sum/1 -> Gain/1
  Idc_n/1 -> Sum/2
  Idc_p/1 -> Sum/1

== system HVDC_VSC_1CPUcore_dcpl/SM_HVDC_VSC/VSC Controller (Station 1)/Discrete VSC Controller (Station 1)/Signal Calculations/DC_Voltage ==
  note: DC Voltage Calculation
  Udc_p : Inport
  Udc_n : Inport  Port=2
  Gain : Gain  Gain=0.5  SaturateOnIntegerOverflow=on  OutDataTypeStr=Inherit: Same as input  ParamDataTypeStr=Inherit: Same as input
  Sum : Sum  Inputs=+-  SaturateOnIntegerOverflow=on
  Udc_meas : Outport
  wires:
  Udc_p/1 -> Sum/1
  Sum/1 -> Gain/1
  Gain/1 -> Udc_meas/1
  Udc_n/1 -> Sum/2

== system HVDC_VSC_1CPUcore_dcpl/SM_HVDC_VSC/VSC Controller (Station 1)/Discrete VSC Controller (Station 1)/Signal Calculations/Filter_Bus_Voltage ==
  note: Filter Bus Voltage Calculation
  Uf_AB : Inport
  Math Function : Math  Operator=magnitude^2  SaturateOnIntegerOverflow=on
  Math Function1 : Math  Operator=sqrt  SaturateOnIntegerOverflow=on
  Sum : Sum  Inputs=+  SaturateOnIntegerOverflow=on
  Uf_meas : Outport
  wires:
  Math Function1/1 -> Uf_meas/1
  Sum/1 -> Math Function1/1
  Math Function/1 -> Sum/1
  Uf_AB/1 -> Math Function/1

== system HVDC_VSC_1CPUcore_dcpl/SM_HVDC_VSC/VSC Controller (Station 1)/Discrete VSC Controller (Station 1)/Signal Calculations/Modulation_Index ==
  note: Modulation Index Calculation
  Vref_lim_AB : Inport
  Udc_meas : Inport  Port=2
  Gain1 : Gain  Gain=k_pu2nom_Vdc  SaturateOnIntegerOverflow=on  OutDataTypeStr=Inherit: Same as input  ParamDataTypeStr=Inherit: Same as input
  MAX:10 MIN: 0 : Saturate  UpperLimit=10  LowerLimit=0
  Math Function1 : Math  Operator=magnitude^2  SaturateOnIntegerOverflow=on
  Math Function2 : Math  Operator=sqrt  SaturateOnIntegerOverflow=on
  Product : Product  Inputs=*/  SaturateOnIntegerOverflow=on  OutDataTypeStr=Inherit: Same as first input
  Saturation : Saturate  UpperLimit=1e6  LowerLimit=1e-6
  Sum : Sum  Inputs=+  SaturateOnIntegerOverflow=on
  Mod_index : Outport
  wires:
  Gain1/1 -> Saturation/1
  MAX:10 MIN: 0/1 -> Mod_index/1
  Saturation/1 -> Product/2
  Product/1 -> MAX:10 MIN: 0/1
  Udc_meas/1 -> Gain1/1
  Sum/1 -> Math Function2/1
  Math Function1/1 -> Sum/1
  Math Function2/1 -> Product/1
  Vref_lim_AB/1 -> Math Function1/1

== system HVDC_VSC_1CPUcore_dcpl/SM_HVDC_VSC/VSC Controller (Station 1)/Discrete VSC Controller (Station 1)/Signal Calculations/PCC_Voltage ==
  note: Active Power Calculation
  U_AB : Inport
  Math Function : Math  Operator=magnitude^2  SaturateOnIntegerOverflow=on
  Math Function1 : Math  Operator=sqrt  SaturateOnIntegerOverflow=on
  Sum : Sum  Inputs=+  SaturateOnIntegerOverflow=on
  Upcc : Outport
  wires:
  U_AB/1 -> Math Function/1
  Math Function/1 -> Sum/1
  Sum/1 -> Math Function1/1
  Math Function1/1 -> Upcc/1

== system HVDC_VSC_1CPUcore_dcpl/SM_HVDC_VSC/VSC Controller (Station 1)/Discrete VSC Controller (Station 1)/Signal Calculations/Reactive_Power ==
  note: Reactive Power Calculation
  U_AB : Inport
  I_AB : Inport  Port=2
  Demux : Demux  Outputs=2
  Demux1 : Demux  Outputs=2
  Product : Product  SaturateOnIntegerOverflow=on  OutDataTypeStr=Inherit: Same as first input
  Product1 : Product  SaturateOnIntegerOverflow=on  OutDataTypeStr=Inherit: Same as first input
  Sum : Sum  Inputs=+-  SaturateOnIntegerOverflow=on
  Qpcc : Outport
  wires:
  Sum/1 -> Qpcc/1
  Product1/1 -> Sum/2
  Product/1 -> Sum/1
  I_AB/1 -> Demux1/1
  U_AB/1 -> Demux/1
  Demux/2 -> Product/2
  Demux1/1 -> Product/1
  Demux/1 -> Product1/1
  Demux1/2 -> Product1/2

== system HVDC_VSC_1CPUcore_dcpl/SM_HVDC_VSC/VSC Controller (Station 1)/Discrete VSC Controller (Station 1)/dq  Transformations/ab0_to_dq0 ==
  note: X0 = X0
  note: Alpha-Beta-zero to dq0
  note: Xd = Xa*sin(wt) - Xb*cos(wt)
  note: Xq = Xa*cos(wt) + Xb*sin(wt)
  ab0 : Inport
  sin_cos : Inport  Port=2
  Demux : Demux  Outputs=2
  Demux1 : Demux  Outputs=3
  Gain3 : Gain  Gain=-1  SaturateOnIntegerOverflow=on  OutDataTypeStr=Inherit: Same as input  ParamDataTypeStr=Inherit: Same as input
  Mux : Mux  Inputs=3
  Product{,1..3} (4 alike) : Product  SaturateOnIntegerOverflow=on  InputSameDT=on  OutDataTypeStr=Inherit: Same as first input
  Sum1 : Sum  Inputs=2  SaturateOnIntegerOverflow=on  InputSameDT=on  OutDataTypeStr=Inherit: Same as first input
  Sum4 : Sum  Inputs=2  SaturateOnIntegerOverflow=on  InputSameDT=on  OutDataTypeStr=Inherit: Same as first input
  dq0 : Outport
  wires:
  Demux1/3 -> Mux/3
  ab0/1 -> Demux1/1
  Mux/1 -> dq0/1
  Product3/1 -> Sum1/2
  Product2/1 -> Sum1/1
  Product1/1 -> Sum4/1
  Demux1/2 -> Product3/1, Product1/1
  Demux/1 -> Product1/2, Product2/2
  Product/1 -> Sum4/2
  Demux1/1 -> Product2/1, Product/1
  Demux/2 -> Product/2, Gain3/1
  sin_cos/1 -> Demux/1
  Sum1/1 -> Mux/1
  Gain3/1 -> Product3/2
  Sum4/1 -> Mux/2

== system HVDC_VSC_1CPUcore_dcpl/SM_HVDC_VSC/VSC Controller (Station 1)/Discrete VSC Controller (Station 1)/dq  Transformations/ab0_to_dq0    ==
  note: Xq = Xa*cos(wt) + Xb*sin(wt)
  note: Xd = Xa*sin(wt) - Xb*cos(wt)
  note: Alpha-Beta-zero to dq0
  note: X0 = X0
  ab0 : Inport
  sin_cos : Inport  Port=2
  Demux : Demux  Outputs=2
  Demux1 : Demux  Outputs=3
  Gain3 : Gain  Gain=-1  SaturateOnIntegerOverflow=on  OutDataTypeStr=Inherit: Same as input  ParamDataTypeStr=Inherit: Same as input
  Mux : Mux  Inputs=3
  Product{,1..3} (4 alike) : Product  SaturateOnIntegerOverflow=on  InputSameDT=on  OutDataTypeStr=Inherit: Same as first input
  Sum1 : Sum  Inputs=2  SaturateOnIntegerOverflow=on  InputSameDT=on  OutDataTypeStr=Inherit: Same as first input
  Sum4 : Sum  Inputs=2  SaturateOnIntegerOverflow=on  InputSameDT=on  OutDataTypeStr=Inherit: Same as first input
  dq0 : Outport
  wires:
  Sum4/1 -> Mux/2
  Gain3/1 -> Product3/2
  Sum1/1 -> Mux/1
  sin_cos/1 -> Demux/1
  Demux/2 -> Gain3/1, Product/2
  Demux1/1 -> Product/1, Product2/1
  Product/1 -> Sum4/2
  Demux/1 -> Product2/2, Product1/2
  Demux1/2 -> Product1/1, Product3/1
  Product1/1 -> Sum4/1
  Product2/1 -> Sum1/1
  Product3/1 -> Sum1/2
  Mux/1 -> dq0/1
  ab0/1 -> Demux1/1
  Demux1/3 -> Mux/3

== system HVDC_VSC_1CPUcore_dcpl/SM_HVDC_VSC/VSC Controller (Station 2)/Discrete VSC Controller (Station 2)/Clark Transformations/CLARK  ==
  note: CLARK transformation
  abc : Inport
  Fcn1 : Fcn  Expr=1/sqrt(3)*(u[2] - u[3])
  Fcn2 : Fcn  Expr=1/3*(2*u[1] - u[2] - u[3])
  Fcn3 : Fcn  Expr=1/3*(u[1] + u[2] + u[3])
  Mux : Mux  Inputs=3
  AB0 : Outport
  wires:
  Fcn2/1 -> Mux/1
  abc/1 -> Fcn1/1, Fcn3/1, Fcn2/1
  Fcn1/1 -> Mux/2
  Fcn3/1 -> Mux/3
  Mux/1 -> AB0/1

== system HVDC_VSC_1CPUcore_dcpl/SM_HVDC_VSC/VSC Controller (Station 2)/Discrete VSC Controller (Station 2)/Clark Transformations/CLARK   ==
  note: CLARK transformation
  abc : Inport
  Fcn1 : Fcn  Expr=1/sqrt(3)*(u[2] - u[3])
  Fcn2 : Fcn  Expr=1/3*(2*u[1] - u[2] - u[3])
  Fcn3 : Fcn  Expr=1/3*(u[1] + u[2] + u[3])
  Mux : Mux  Inputs=3
  AB0 : Outport
  wires:
  Mux/1 -> AB0/1
  Fcn3/1 -> Mux/3
  Fcn1/1 -> Mux/2
  abc/1 -> Fcn2/1, Fcn3/1, Fcn1/1
  Fcn2/1 -> Mux/1

== system HVDC_VSC_1CPUcore_dcpl/SM_HVDC_VSC/VSC Controller (Station 2)/Discrete VSC Controller (Station 2)/Clark Transformations/CLARK_YD ==
  note: Rotation of pi/6
  note: Rotation of - pi/6
  note: Transformer Connexion:
      | YY = 0
      | YD1 (laging) = 1
      | YD11 (leading)= 2
  note: CLARK transformation
  abc : Inport
  Tr_conx : Inport  Port=2
  CLARK : Subsystem  AncestorBlock=lib_mesures/CLARK  TreatAsAtomicUnit=on
  CLARK_YD1 : Subsystem  AncestorBlock=lib_mesures/CLARK  TreatAsAtomicUnit=on
  CLARK_YD11 : Subsystem  AncestorBlock=lib_mesures/CLARK  TreatAsAtomicUnit=on
  Constant : Constant  Value=2
  Constant1 : Constant  Value=0
  Constant2 : Constant
  Relational Operator1 : RelationalOperator  Operator===  InputSameDT=on
  Relational Operator2 : RelationalOperator  Operator===  InputSameDT=on
  Relational Operator3 : RelationalOperator  Operator===  InputSameDT=on
  Sum : Sum  Inputs=+++  SaturateOnIntegerOverflow=on
  AB0 : Outport
  wires:
  Constant2/1 -> Relational Operator3/2
  Relational Operator2/1 -> CLARK/Enable
  Constant1/1 -> Relational Operator2/2
  CLARK/1(AB0) -> Sum/3
  Sum/1 -> AB0/1
  CLARK_YD1/1(AB0) -> Sum/2
  CLARK_YD11/1(AB0) -> Sum/1
  abc/1 -> CLARK/1(abc), CLARK_YD1/1(abc), CLARK_YD11/1(abc)
  Relational Operator1/1 -> CLARK_YD11/Enable
  Relational Operator3/1 -> CLARK_YD1/Enable
  Tr_conx/1 -> Relational Operator3/1, Relational Operator2/1, Relational Operator1/1
  Constant/1 -> Relational Operator1/2

== system HVDC_VSC_1CPUcore_dcpl/SM_HVDC_VSC/VSC Controller (Station 2)/Discrete VSC Controller (Station 2)/Clark Transformations/CLARK_YD  ==
  note: CLARK transformation
  note: Transformer Connexion:
      | YY = 0
      | YD1 (laging) = 1
      | YD11 (leading)= 2
  note: Rotation of - pi/6
  note: Rotation of pi/6
  abc : Inport
  Tr_conx : Inport  Port=2
  CLARK : Subsystem  AncestorBlock=lib_mesures/CLARK  TreatAsAtomicUnit=on
  CLARK_YD1 : Subsystem  AncestorBlock=lib_mesures/CLARK  TreatAsAtomicUnit=on
  CLARK_YD11 : Subsystem  AncestorBlock=lib_mesures/CLARK  TreatAsAtomicUnit=on
  Constant : Constant  Value=2
  Constant1 : Constant  Value=0
  Constant2 : Constant
  Relational Operator1 : RelationalOperator  Operator===  InputSameDT=on
  Relational Operator2 : RelationalOperator  Operator===  InputSameDT=on
  Relational Operator3 : RelationalOperator  Operator===  InputSameDT=on
  Sum : Sum  Inputs=+++  SaturateOnIntegerOverflow=on
  AB0 : Outport
  wires:
  Constant/1 -> Relational Operator1/2
  Tr_conx/1 -> Relational Operator1/1, Relational Operator2/1, Relational Operator3/1
  Relational Operator3/1 -> CLARK_YD1/Enable
  Relational Operator1/1 -> CLARK_YD11/Enable
  abc/1 -> CLARK_YD11/1(abc), CLARK_YD1/1(abc), CLARK/1(abc)
  CLARK_YD11/1(AB0) -> Sum/1
  CLARK_YD1/1(AB0) -> Sum/2
  Sum/1 -> AB0/1
  CLARK/1(AB0) -> Sum/3
  Constant1/1 -> Relational Operator2/2
  Relational Operator2/1 -> CLARK/Enable
  Constant2/1 -> Relational Operator3/2

== system HVDC_VSC_1CPUcore_dcpl/SM_HVDC_VSC/VSC Controller (Station 2)/Discrete VSC Controller (Station 2)/DC Voltage Balance Control/Regulator ==
  note: Reset states when enabling
  note: Voltage Sign
  note: Reversed Current Sign
  V_ref_lim_abc : Inport
  Iv_abc : Inport  Port=2
  Udc_0_mean : Inport  Port=3
  Enable : EnablePort  StatesWhenEnabling=reset
  Constant1 : Constant  Value=0
  Constant13 : Constant  Value=Ki_dcvbc
  Constant2 : Constant  Value=0
  Constant3 : Constant  Value=-1
  Constant4 : Constant
  Constant5 : Constant
  Constant6 : Constant  Value=-1
  Constant7 : Constant  Value=0
  Constant8 : Constant  Value=Kp_dcvbc
  "PI_regulator " : Subsystem  mask(PI regulator - type 2){max_i=max_out_dcvbc, min_i=min_out_dcvbc, i_ic=0, max_out=max_out_dcvbc, min_out=min_out_dcvbc, Ts=Ts_Control}
      mask prompts: max_i "Integrator maximum  limit:"; min_i "Integrator minimum  limit:"; i_ic "Integrator initial condition:"; max_out "Output maximum limit:"; min_out "Output minimum limit:"; Ts "Sample time: (s)"
  Product : Product  Inputs=3  SaturateOnIntegerOverflow=on  OutDataTypeStr=Inherit: Same as first input
  Relational Operator : RelationalOperator  Operator=<
  Relational Operator1 : RelationalOperator  Operator=<
  Switch : Switch  Threshold=0.5  SaturateOnIntegerOverflow=on
  Switch1 : Switch  Threshold=0.5  SaturateOnIntegerOverflow=on
  dV_ref_abc_dcvbc : Outport
  wires:
  Switch1/1 -> Product/2
  Constant1/1 -> "PI_regulator "/5(Kf), "PI_regulator "/2(Meas)
  Constant13/1 -> "PI_regulator "/3(Ki)
  Constant8/1 -> "PI_regulator "/4(Kp)
  "PI_regulator "/1(Out) -> Product/3
  Constant2/1 -> Relational Operator/2
  Constant3/1 -> Switch/1
  Constant4/1 -> Switch/3
  Relational Operator/1 -> Switch/2
  Constant5/1 -> Switch1/1
  Constant6/1 -> Switch1/3
  Relational Operator1/1 -> Switch1/2
  Switch/1 -> Product/1
  V_ref_lim_abc/1 -> Relational Operator/1
  Product/1 -> dV_ref_abc_dcvbc/1
  Iv_abc/1 -> Relational Operator1/1
  Udc_0_mean/1 -> "PI_regulator "/1(Ord)
  Constant7/1 -> Relational Operator1/2
